simulink model "mConfigBlk"  (R2019b)
settings: configuration reference "ConfigSetDesktopFixedStep" (kept outside this file)
libraries: autolibshared x1, VsrLibMdlConfig x1
settings Model: DataDictionary=TestDataDictionary.sldd  Creator=9bt  LastModifiedBy=4qz
settings ConfigSetRef: SourceName=ConfigSetDesktopFixedStep

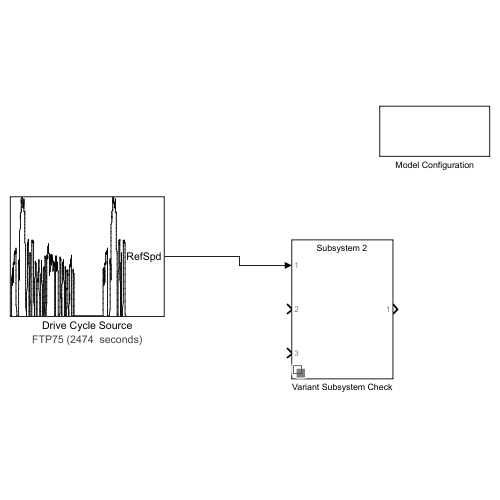
[thumbnail: Simulink's stored preview of the top-level diagram]
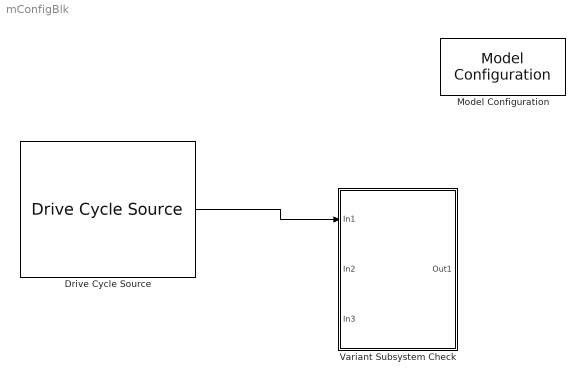
== system mConfigBlk ==
  Drive Cycle Source : autolibshared/Drive Cycle Source  cycleVar=FTP75  fileVar=cycleFTP75.mat  tfinal="2474  seconds"  cycleRepeat=off  outAccPort=off  outGearPort=off  gearList=No gear data  t_wot1=5  xdot_woto=0  xdot_wot1=30  t_wot2=20  xdot_wot2=0  t_wotend=30  srcUnit=m/s  outUnit=m/s  srcAccUnit=m/s/s  outAccUnit=m/s^2  dt=0  aMode=1
  Model Configuration : VsrLibMdlConfig/Model Configuration  ConfigFileName=getTestConfigs
  Variant Subsystem Check : Subsystem  Variant=on  VariantControlMode=label  LabelModeActiveChoice=Choice_2
  wires:
  Drive Cycle Source/1 -> Variant Subsystem Check/1(In1)

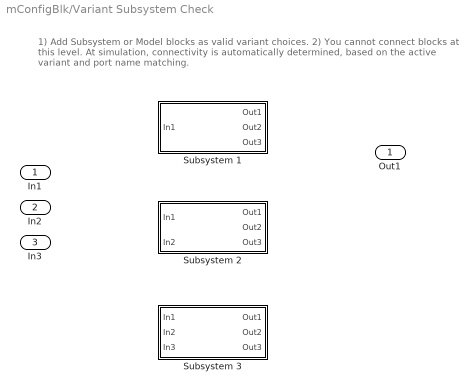
== system mConfigBlk/Variant Subsystem Check ==
  note: 1) Add Subsystem or Model blocks as valid variant choices.
      | 2) You cannot connect blocks at this level. At simulation, connectivity is automatically
      | determined, based on the active variant and port name matching.
  In1 : Inport
  In2 : Inport  Port=2
  In3 : Inport  Port=3
  Subsystem 1 : Subsystem  VariantControl=Choice_1
  Subsystem 2 : Subsystem  VariantControl=Choice_2
  Subsystem 3 : Subsystem  VariantControl=Choice_3
  Out1 : Outport

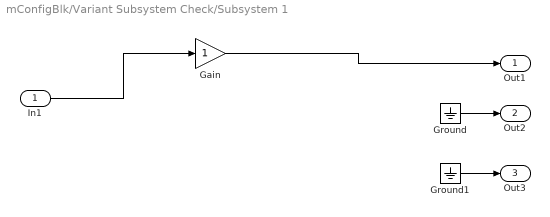
== system mConfigBlk/Variant Subsystem Check/Subsystem 1 ==
  In1 : Inport
  Gain : Gain
  Ground : Ground
  Ground1 : Ground
  Out1 : Outport
  Out2 : Outport  Port=2
  Out3 : Outport  Port=3
  wires:
  Ground1/1 -> Out3/1
  Ground/1 -> Out2/1
  Gain/1 -> Out1/1
  In1/1 -> Gain/1

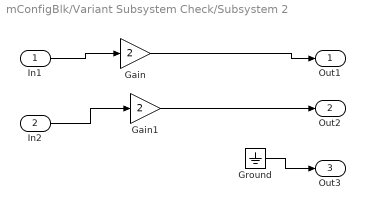
== system mConfigBlk/Variant Subsystem Check/Subsystem 2 ==
  In1 : Inport
  In2 : Inport  Port=2
  Gain : Gain  Gain=2
  Gain1 : Gain  Gain=2
  Ground : Ground
  Out1 : Outport
  Out2 : Outport  Port=2
  Out3 : Outport  Port=3
  wires:
  Ground/1 -> Out3/1
  In2/1 -> Gain1/1
  In1/1 -> Gain/1
  Gain/1 -> Out1/1
  Gain1/1 -> Out2/1

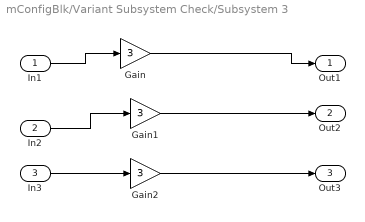
== system mConfigBlk/Variant Subsystem Check/Subsystem 3 ==
  In1 : Inport
  In2 : Inport  Port=2
  In3 : Inport  Port=3
  Gain : Gain  Gain=3
  Gain1 : Gain  Gain=3
  Gain2 : Gain  Gain=3
  Out1 : Outport
  Out2 : Outport  Port=2
  Out3 : Outport  Port=3
  wires:
  In3/1 -> Gain2/1
  In1/1 -> Gain/1
  Gain2/1 -> Out3/1
  Gain/1 -> Out1/1
  Gain1/1 -> Out2/1
  In2/1 -> Gain1/1
